simulink model "Controle_Adaptativo_1"  (R2024b)
settings: Solver=FixedStepAuto  StartTime=0.0  StopTime=5  FixedStep=0.001  RelTol=1e-3
InitFcn:
  | %Massa Verdadeira
  | m = 2;
  | 
  | %Estimativa Inicial da massa
  | mh0 =0.5;
  | 
  | %Parâmetros do Controlador PD
  | Kp = 100;
  | Kd = 20;
  | 
  | %Parâmetros da Lei de Aprendizagem
  | Gamma = 5;
settings Model: Creator=IDRZBOOK002  LastModifiedBy=IDRZBOOK002

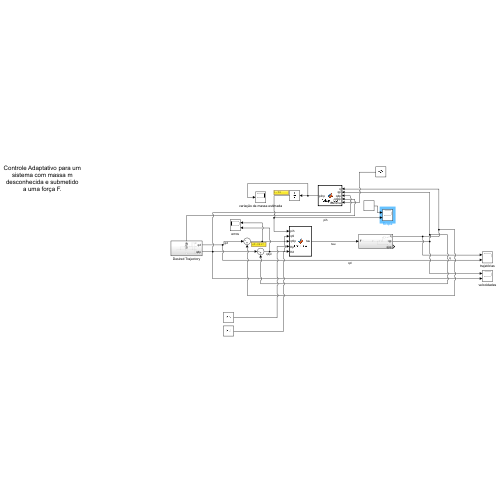
[thumbnail: Simulink's stored preview of the top-level diagram]
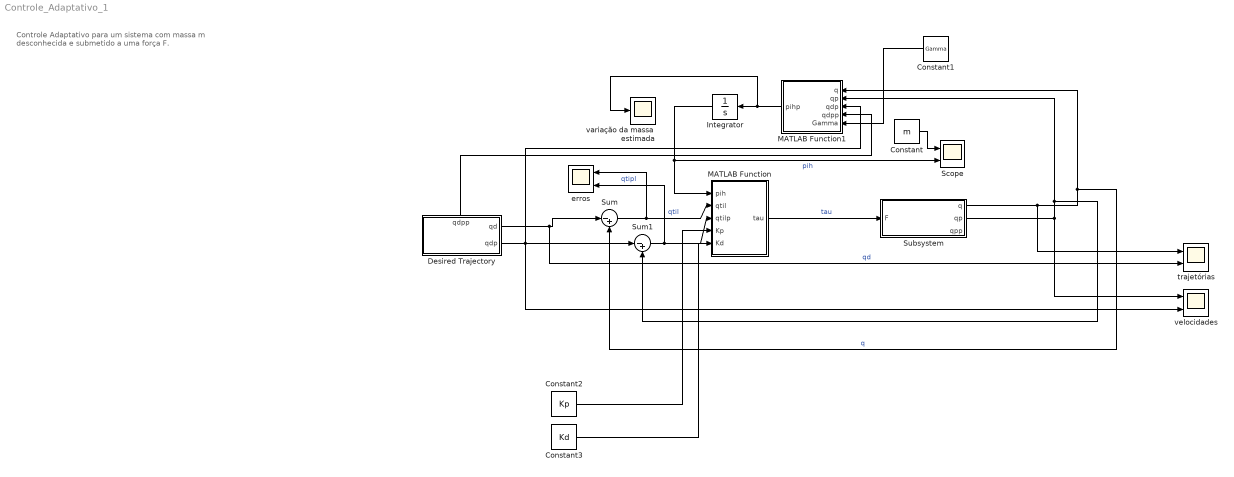
== system Controle_Adaptativo_1 ==
  note: Controle Adaptativo para um sistema com massa m desconhecida e submetido a uma força F.
  Constant : Constant  Value=m
  Constant1 : Constant  Value=Gamma
  Constant2 : Constant  Value=Kp
  Constant3 : Constant  Value=Kd
  Desired Trajectory : Subsystem
      settings: PortSchema="{\"entries\":[{\"content\":{\"sides\":[{\"content\":{},\"type\":\"ConnectorPlacement.EquallySpacedRectSide\",\"uuid\":\"fde9c678-b2f0-48bb-8b77-059617d4abcd\"},{\"content\":{\"connectorIds\":[\"Out1\",\"Out2\"],\"side\":\"RIGHT\"},\"type\":\"ConnectorPlacement.EquallySpacedRectSide\",\"uuid\":\"217a379d-a803-41b8-8b57-bfab0073b449\"},{\"content\":{\"connectorIds\":[\"Out3\"],\"side\":\"TOP\"},\"type\":\"ConnectorPlacement.EquallySpacedRectSide\",\"uuid\":\"f11199d7-3a24-4232-8e20-31e0b008a8a8\"}]},\"type\":\"ConnectorPlacement.EquallySpacedConnector\",\"uuid\":\"b1296899-b312-4960-bb2e-673c4701805b\"}],\"packageUris\":[\"http://schema.mathworks.com/mf0/Connector/R2020b\"],\"version\":\"1.0\"}"
  Integrator : Integrator  InitialCondition=mh0
  MATLAB Function : MATLAB Function  TreatAsAtomicUnit=on
  MATLAB Function1 : MATLAB Function  TreatAsAtomicUnit=on
  Scope : Scope  NumInputPorts=2
  Subsystem : Subsystem
  Sum : Sum  Inputs=|-+
  Sum1 : Sum  Inputs=|-+
  erros : Scope  NumInputPorts=2
  trajetórias : Scope  NumInputPorts=2
  variação da massa estimada : Scope
  velocidades : Scope  NumInputPorts=2
  wires:
  Desired Trajectory/1(qd) -> trajetórias/2, Sum/1  "qd"
  MATLAB Function/1(tau) -> Subsystem/1(F)  "tau"
  Sum/1 -> erros/1, MATLAB Function/2(qtil)  "qtil"
  Sum1/1 -> MATLAB Function/3(qtilp), erros/2  "qtipl"
  Subsystem/1(q) -> trajetórias/1, MATLAB Function1/1(q), Sum/2  "q"
  Subsystem/2(qp) -> velocidades/1, MATLAB Function1/2(qp), Sum1/2
  Desired Trajectory/2(qdp) -> velocidades/2, MATLAB Function1/3(qdp), Sum1/1
  MATLAB Function1/1(pihp) -> variação da massa estimada/1, Integrator/1
  Integrator/1 -> MATLAB Function/1(pih), Scope/2  "pih"
  Desired Trajectory/3(qdpp) -> MATLAB Function1/4(qdpp)
  Constant/1 -> Scope/1
  Constant1/1 -> MATLAB Function1/5(Gamma)
  Constant2/1 -> MATLAB Function/4(Kp)
  Constant3/1 -> MATLAB Function/5(Kd)

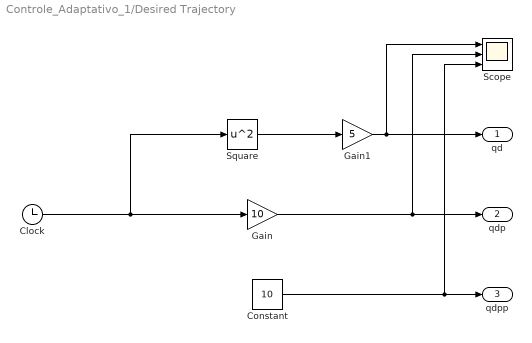
== system Controle_Adaptativo_1/Desired Trajectory ==
  Clock : Clock
  Constant : Constant  Value=10
  Gain : Gain  Gain=10
  Gain1 : Gain  Gain=5
  Scope : Scope  NumInputPorts=3
  Square : Math  Operator=square
  qd : Outport
  qdp : Outport  Port=2
  qdpp : Outport  Port=3
  wires:
  Clock/1 -> Square/1, Gain/1
  Gain/1 -> Scope/2, qdp/1
  Constant/1 -> Scope/3, qdpp/1
  Gain1/1 -> Scope/1, qd/1
  Square/1 -> Gain1/1

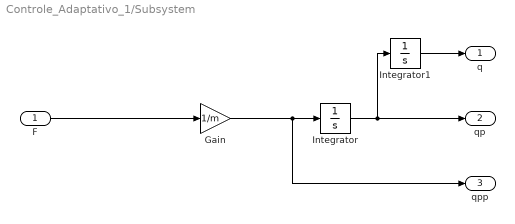
== system Controle_Adaptativo_1/Subsystem ==
  F : Inport
  Gain : Gain  Gain=1/m
  Integrator : Integrator
  Integrator1 : Integrator  InitialCondition=0.5
  q : Outport
  qp : Outport  Port=2
  qpp : Outport  Port=3
  wires:
  F/1 -> Gain/1
  Gain/1 -> Integrator/1, qpp/1
  Integrator/1 -> Integrator1/1, qp/1
  Integrator1/1 -> q/1

== matlab function Controle_Adaptativo_1/MATLAB Function1 ==
  data: q input; pihp output; qp input; qdp input; qdpp input; Gamma input
function pihp = Adapt_law(q,qp,qdp,qdpp, Gamma)
Y = [10];
pihp = -Gamma^-1*Y*(qp-qdp);

== matlab function Controle_Adaptativo_1/MATLAB Function ==
  data: pih input; tau output; qtil input; qtilp input; Kp input; Kd input
function tau = Ctr_Law(pih,qtil,qtilp, Kp, Kd)
Y = 10;
tau = Y*pih-Kp*(qtil)-Kd*qtilp;
